simulink model "sampleModel1965_5"  (R2023a)
settings: Solver=VariableStepAuto  StartTime=0.0  StopTime=10.0  RelTol=1e-3
libraries: simulink x2, hdlsllib x2
settings Model: Creator=user1  LastModifiedBy=user1

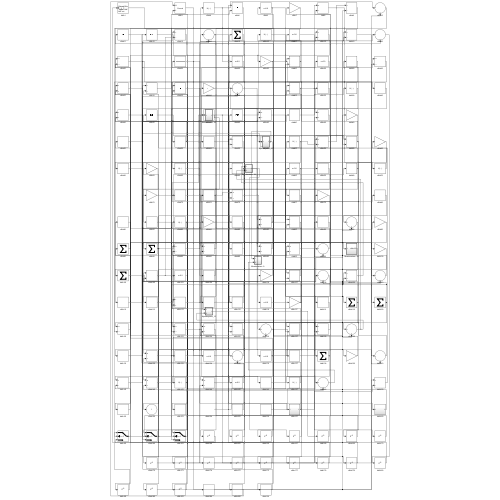
[thumbnail: Simulink's stored preview of the top-level diagram]
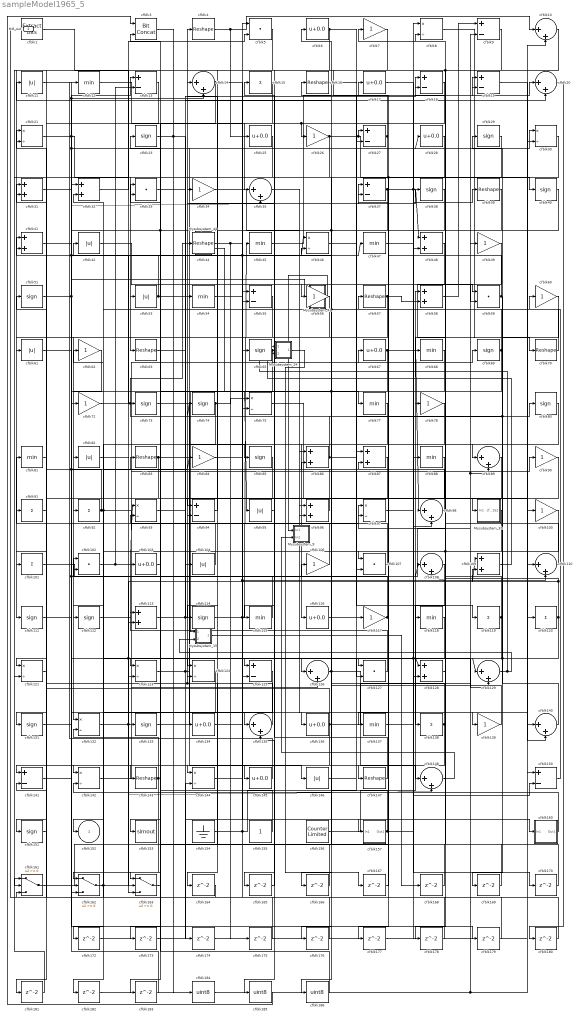
== system sampleModel1965_5 ==
  Mysubsystem_15 : Subsystem  TreatAsAtomicUnit=on  RTWFcnName=Mysubsystem_15
      settings: RTWFcnNameOpts=User specified  RTWFileNameOpts=Use function name
  Mysubsystem_24 : Subsystem  TreatAsAtomicUnit=on  RTWFcnName=Mysubsystem_24
      settings: RTWFcnNameOpts=User specified  RTWFileNameOpts=Use function name
  Mysubsystem_32 : Subsystem  TreatAsAtomicUnit=on  RTWFcnName=Mysubsystem_32
      settings: RTWFcnNameOpts=User specified  RTWFileNameOpts=Use function name
  Mysubsystem_41 : Subsystem  TreatAsAtomicUnit=on  RTWFcnName=Mysubsystem_41
      settings: RTWFcnNameOpts=User specified  RTWFileNameOpts=Use function name
  Mysubsystem_44 : Subsystem  TreatAsAtomicUnit=on  RTWFcnName=Mysubsystem_44
      settings: RTWFcnNameOpts=User specified  RTWFileNameOpts=Use function name
  Mysubsystem_9 : Subsystem  TreatAsAtomicUnit=on  RTWFcnName=Mysubsystem_9
      settings: RTWFcnNameOpts=User specified  RTWFileNameOpts=Use function name
  cfblk1 : simulink/Logic and Bit Operations/Extract Bits  bitsToExtract=Upper half  numBits=8  bitIdxRange=[0 7]  outScalingMode=Preserve fixed-point scaling
      settings: LibrarySourceBlock=|
      | hdlsllib/Logic and Bit
      | Operations/Extract Bits
  cfblk{10,14,20,35,89,98,108,110,126,129,135,140,148} (13 alike) : Sum  Inputs=|++  OutDataTypeStr=uint8
  cfblk{7,26,34,49,56,60,62,72,78,84,90,100,106,117,139} (15 alike) : Gain  OutDataTypeStr=uint8
  cfblk{15,91..92,101,119..120,138} (7 alike) : Sum  Inputs=+  OutDataTypeStr=uint8
  cfblk{5,33,59,102,107,127} (6 alike) : DotProduct  OutDataTypeStr=uint8
  cfblk{6,17,25,28,67,103,116,134,136,145} (10 alike) : Bias  Bias=0.0  SaturateOnIntegerOverflow=off
  cfblk{11,42,53,61,82,95,104,146} (8 alike) : Abs  OutDataTypeStr=uint8  SaturateOnIntegerOverflow=off
  cfblk{31..32,41,48,58,86..87,96,109,113,128} (11 alike) : Sum  OutDataTypeStr=uint8
  cfblk{23,29,38,40,51,65,69,73..74,80,85,111..112,114,131,133,151} (17 alike) : Signum
  cfblk{12,45,47,54,68,77,81,88,115,118,137} (11 alike) : MinMax  OutDataTypeStr=uint8
  cfblk{8,21,30,46,75,93,97,121,123..124,132,142,144} (13 alike) : Product  Inputs=*/  OutDataTypeStr=uint8  RndMeth=Zero  SaturateOnIntegerOverflow=on
  cfblk{9,13,18..19,27,37,55,94,125,141,150} (11 alike) : Sum  Inputs=+-  OutDataTypeStr=uint8
  cfblk{4,16,39,44,57,63,70,83,143,147} (10 alike) : Reshape
  cfblk153 : ToWorkspace  VariableName=simout  SaveFormat=Timeseries  SampleTime=-1
  cfblk154 : Ground
  cfblk155 : Constant  OutDataTypeStr=uint8  SampleTime=-1
  cfblk156 : hdlsllib/Sources/Counter Limited  uplimit=7  tsamp=-1
  cfblk157 : Subsystem
      settings: LibrarySourceBlock=|
      | hdlsllib/Ports &
      | Subsystems/Subsystem
  cfblk160 : Subsystem
      settings: LibrarySourceBlock=|
      | hdlsllib/Ports &
      | Subsystems/Subsystem
  cfblk161 : Switch  OutDataTypeStr=uint8  SaturateOnIntegerOverflow=off  InputSameDT=off
  cfblk162 : Switch  OutDataTypeStr=uint8  SaturateOnIntegerOverflow=off  InputSameDT=off
  cfblk163 : Switch  OutDataTypeStr=uint8  SaturateOnIntegerOverflow=off  InputSameDT=off
  cfblk{164..170,172..183} (19 alike) : Delay  SampleTime=1
  cfblk184 : DataTypeConversion  OutDataTypeStr=uint8  SaturateOnIntegerOverflow=off  RndMeth=Floor
  cfblk185 : DataTypeConversion  OutDataTypeStr=uint8  SaturateOnIntegerOverflow=off  RndMeth=Floor
  cfblk186 : DataTypeConversion  OutDataTypeStr=uint8  SaturateOnIntegerOverflow=off  RndMeth=Floor
  cfblk3 : hdlsllib/Logic and Bit Operations/Bit Concat  numInputs=2
  cfblk152 : Outport  OutDataTypeStr=uint8  VectorParamsAs1DForOutWhenUnconnected=off
  Hdl_out : Outport  Port=2  OutDataTypeStr=uint8
  wires:
  cfblk65/1 -> cfblk139/1, cfblk183/1
  cfblk42/1 -> cfblk56/1
  cfblk73/1 -> cfblk135/1
  cfblk77/1 -> cfblk116/1
  cfblk92/1 -> cfblk69/1, cfblk162/1, cfblk21/2
  cfblk58/1 -> cfblk9/1
  cfblk48/1 -> cfblk70/1
  cfblk53/1 -> cfblk37/1, cfblk31/2
  cfblk157/1(Out1) -> cfblk16/1, cfblk150/2
  cfblk145/1 -> cfblk12/1
  cfblk114/1 -> cfblk45/1, cfblk67/1
  cfblk150/1 -> cfblk60/1
  cfblk161/1 -> cfblk147/1
  cfblk110/1 -> cfblk7/1
  cfblk4/1 -> cfblk10/1, cfblk25/1
  cfblk112/1 -> cfblk90/1
  cfblk27/1 -> cfblk111/1, cfblk75/2
  cfblk86/1 -> Mysubsystem_44/1(In1), cfblk73/1, cfblk80/1
  cfblk14/1 -> cfblk129/2, cfblk173/1
  cfblk8/1 -> cfblk100/1
  cfblk56/1 -> cfblk132/1
  cfblk133/1 -> cfblk30/1
  cfblk118/1 -> cfblk142/1
  cfblk87/1 -> cfblk92/1
  cfblk141/1 -> cfblk47/1, cfblk35/2, cfblk84/1, cfblk108/1
  cfblk3/1 -> cfblk184/1
  cfblk115/1 -> cfblk102/1
  cfblk123/1 -> cfblk146/1, cfblk160/1(In1)
  cfblk39/1 -> cfblk115/1
  cfblk98/1 -> cfblk42/1
  cfblk35/1 -> cfblk96/1
  cfblk143/1 -> cfblk132/2, cfblk172/1
  cfblk28/1 -> cfblk126/1, cfblk177/1
  cfblk135/1 -> cfblk4/1, cfblk31/1
  cfblk19/1 -> cfblk120/1
  cfblk147/1 -> cfblk34/1
  cfblk29/1 -> cfblk63/1
  cfblk121/1 -> cfblk41/1
  cfblk75/1 -> cfblk110/1
  cfblk18/1 -> cfblk26/1, cfblk164/1
  cfblk62/1 -> cfblk82/1
  cfblk162/1 -> cfblk62/1, cfblk109/2
  cfblk156/1 -> cfblk58/1
  cfblk108/1 -> cfblk138/1
  cfblk13/1 -> cfblk101/1
  cfblk81/1 -> cfblk141/1
  cfblk101/1 -> cfblk106/1
  cfblk30/1 -> cfblk53/1
  cfblk45/1 -> cfblk19/1
  cfblk57/1 -> cfblk131/1, cfblk58/2
  cfblk132/1 -> cfblk97/1, cfblk148/2
  cfblk131/1 -> cfblk72/1
  cfblk6/1 -> cfblk119/1, cfblk163/2
  cfblk85/1 -> cfblk121/1
  cfblk74/1 -> cfblk112/1, cfblk75/1
  cfblk129/1 -> Mysubsystem_24/2(In2), Mysubsystem_15/2(In2)
  cfblk67/1 -> cfblk98/1, cfblk107/2
  cfblk21/1 -> cfblk113/2, cfblk179/1
  cfblk26/1 -> cfblk27/1, cfblk140/1, cfblk121/2
  cfblk142/1 -> cfblk126/2
  cfblk51/1 -> cfblk123/1, cfblk46/2
  cfblk70/1 -> cfblk32/2, cfblk6/1
  cfblk40/1 -> cfblk125/1
  cfblk9/1 -> cfblk61/1, cfblk178/1
  cfblk88/1 -> cfblk151/1
  cfblk11/1 -> Mysubsystem_41/1(In1), cfblk14/2
  cfblk68/1 -> cfblk95/1, cfblk166/1
  cfblk49/1 -> cfblk68/1
  cfblk128/1 -> cfblk78/1
  cfblk120/1 -> cfblk8/2, cfblk109/1, cfblk127/2
  cfblk72/1 -> cfblk44/1
  cfblk7/1 -> cfblk94/1
  cfblk10/1 -> cfblk145/1
  cfblk94/1 -> cfblk14/1
  cfblk54/1 -> cfblk59/1
  cfblk46/1 -> cfblk87/1
  cfblk83/1 -> cfblk85/1, cfblk162/2
  cfblk160/1(Out1) -> cfblk142/2
  cfblk102/1 -> cfblk93/1, cfblk13/2
  cfblk104/1 -> cfblk81/1
  cfblk78/1 -> cfblk96/2
  cfblk146/1 -> cfblk19/2
  cfblk139/1 -> cfblk41/2
  cfblk103/1 -> cfblk143/1
  cfblk17/1 -> cfblk98/2
  cfblk44/1 -> cfblk59/2, cfblk175/1
  cfblk116/1 -> cfblk117/1
  cfblk89/1 -> cfblk127/1
  cfblk138/1 -> cfblk11/1, cfblk181/1
  cfblk96/1 -> cfblk54/1
  cfblk33/1 -> cfblk104/1
  cfblk84/1 -> cfblk110/2, cfblk157/1(In1)
  cfblk137/1 -> cfblk88/1
  cfblk23/1 -> Mysubsystem_32/1(In1), cfblk134/1
  cfblk59/1 -> cfblk17/1, cfblk89/1
  cfblk5/1 -> cfblk161/2
  cfblk113/1 -> cfblk9/2, cfblk20/2
  cfblk41/1 -> cfblk136/1
  cfblk34/1 -> cfblk86/1
  cfblk126/1 -> cfblk148/1, cfblk176/1
  cfblk37/1 -> cfblk48/1, cfblk40/1, cfblk163/3
  cfblk61/1 -> cfblk28/1, cfblk13/1
  cfblk140/1 -> cfblk74/1, cfblk29/1
  cfblk80/1 -> cfblk114/1
  cfblk15/1 -> cfblk35/1
  cfblk107/1 -> cfblk94/2
  cfblk134/1 -> cfblk65/1
  cfblk119/1 -> cfblk97/2, cfblk137/1
  cfblk154/1 -> cfblk5/1, cfblk27/2
  cfblk117/1 -> cfblk23/1, cfblk87/2
  cfblk25/1 -> cfblk125/2
  cfblk69/1 -> cfblk107/1, cfblk57/1
  cfblk12/1 -> cfblk55/2
  cfblk111/1 -> cfblk83/1
  cfblk106/1 -> cfblk15/1
  cfblk127/1 -> cfblk103/1
  cfblk136/1 -> cfblk144/1, cfblk20/1, cfblk21/1
  cfblk144/1 -> cfblk38/1, cfblk46/1
  cfblk124/1 -> cfblk163/1
  cfblk1/1 -> cfblk133/1
  cfblk82/1 -> cfblk128/1, cfblk128/2, cfblk140/2
  cfblk93/1 -> cfblk18/1
  cfblk91/1 -> cfblk51/1
  cfblk100/1 -> cfblk124/1, cfblk108/2
  cfblk155/1 -> cfblk113/1
  cfblk163/1 -> cfblk33/1
  cfblk32/1 -> cfblk5/2
  cfblk55/1 -> cfblk123/2
  cfblk151/1 -> cfblk91/1
  cfblk16/1 -> cfblk118/1
  cfblk38/1 -> cfblk153/1, cfblk162/3, cfblk186/1
  cfblk31/1 -> cfblk77/1
  cfblk60/1 -> cfblk129/1, cfblk169/1
  cfblk47/1 -> cfblk39/1
  cfblk164/1 -> cfblk1/1
  cfblk95/1 -> cfblk165/1
  cfblk165/1 -> cfblk135/2
  cfblk166/1 -> cfblk93/2
  cfblk167/1 -> cfblk37/2
  cfblk168/1 -> cfblk86/2
  cfblk169/1 -> cfblk18/2
  cfblk97/1 -> cfblk170/1
  cfblk170/1 -> cfblk124/2
  cfblk172/1 -> cfblk144/2
  cfblk173/1 -> cfblk8/1
  cfblk63/1 -> cfblk174/1
  cfblk174/1 -> cfblk10/2
  cfblk175/1 -> cfblk102/2
  cfblk176/1 -> cfblk161/3
  cfblk177/1 -> cfblk48/2
  cfblk178/1 -> cfblk33/2
  cfblk179/1 -> cfblk141/2
  cfblk20/1 -> cfblk180/1
  cfblk180/1 -> cfblk55/1
  cfblk181/1 -> cfblk161/1
  cfblk125/1 -> cfblk182/1
  cfblk182/1 -> cfblk30/2
  cfblk183/1 -> cfblk32/1
  cfblk184/1 -> cfblk89/2, cfblk49/1, cfblk150/1
  cfblk90/1 -> cfblk185/1
  cfblk185/1 -> cfblk3/1
  cfblk186/1 -> cfblk3/2
  cfblk148/1 -> Mysubsystem_9/2(In2)
  Mysubsystem_15/1(Out1) -> cfblk168/1
  cfblk109/1 -> Mysubsystem_24/1(In1)
  Mysubsystem_24/1(Out1) -> cfblk167/1
  Mysubsystem_32/1(cfblk152) -> cfblk152/1
  Mysubsystem_41/1(Out1) -> Mysubsystem_9/1(In1)
  Mysubsystem_44/1(Out1) -> Mysubsystem_15/1(In1)

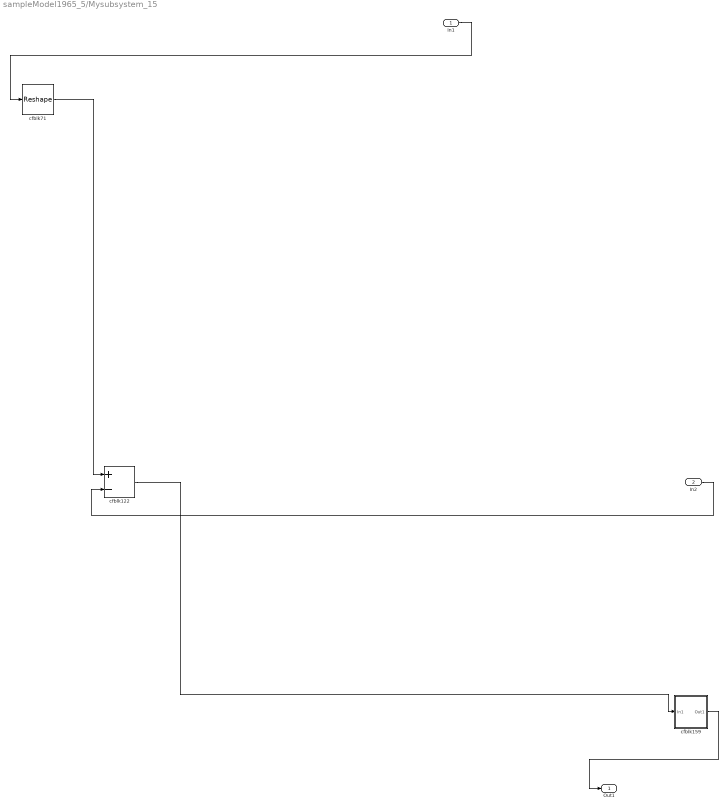
== system sampleModel1965_5/Mysubsystem_15 ==
  In1 : Inport
  In2 : Inport  Port=2
  cfblk122 : Sum  Inputs=+-
  cfblk159 : Subsystem
      settings: LibrarySourceBlock=|
      | hdlsllib/Ports &
      | Subsystems/Subsystem
  cfblk71 : Reshape
  Out1 : Outport
  wires:
  In2/1 -> cfblk122/2
  cfblk71/1 -> cfblk122/1
  cfblk159/1(Out1) -> Out1/1
  cfblk122/1 -> cfblk159/1(In1)
  In1/1 -> cfblk71/1

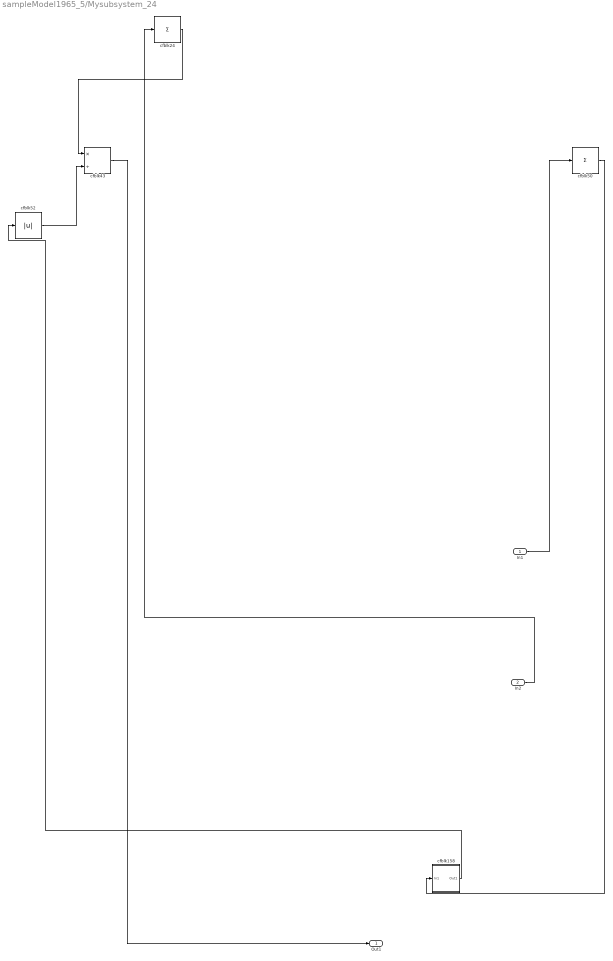
== system sampleModel1965_5/Mysubsystem_24 ==
  In1 : Inport
  In2 : Inport  Port=2
  cfblk158 : Subsystem
      settings: LibrarySourceBlock=|
      | hdlsllib/Ports &
      | Subsystems/Subsystem
  cfblk24 : Sum  Inputs=+
  cfblk43 : Product  Inputs=*/  RndMeth=Zero  SaturateOnIntegerOverflow=on
  cfblk50 : Sum  Inputs=+
  cfblk52 : Abs  SaturateOnIntegerOverflow=off
  Out1 : Outport
  wires:
  cfblk52/1 -> cfblk43/2
  cfblk50/1 -> cfblk158/1(In1)
  In1/1 -> cfblk50/1
  cfblk43/1 -> Out1/1
  cfblk158/1(Out1) -> cfblk52/1
  cfblk24/1 -> cfblk43/1
  In2/1 -> cfblk24/1

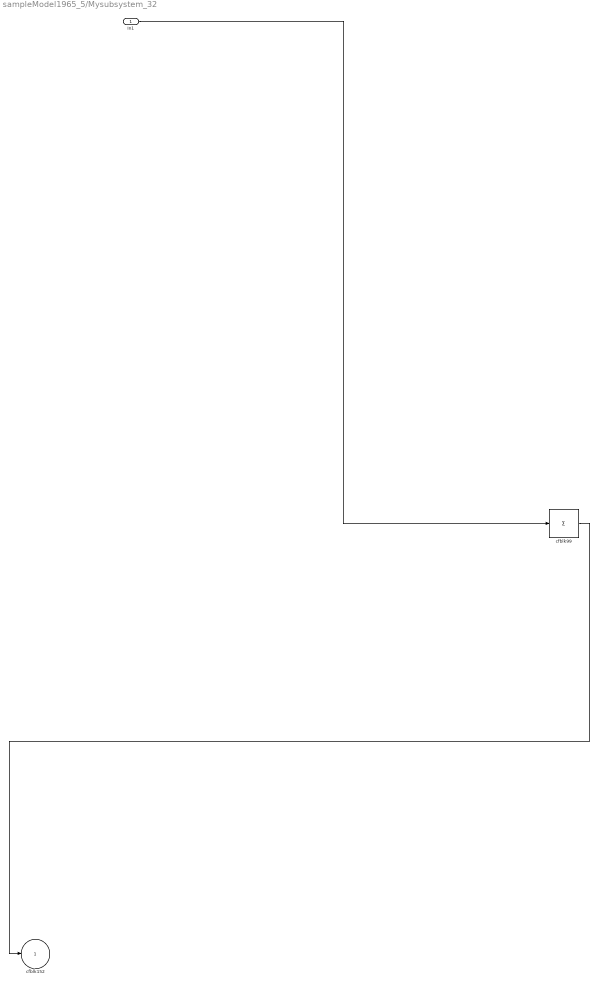
== system sampleModel1965_5/Mysubsystem_32 ==
  In1 : Inport
  cfblk99 : Sum  Inputs=+
  cfblk152 : Outport  VectorParamsAs1DForOutWhenUnconnected=off
  wires:
  cfblk99/1 -> cfblk152/1
  In1/1 -> cfblk99/1

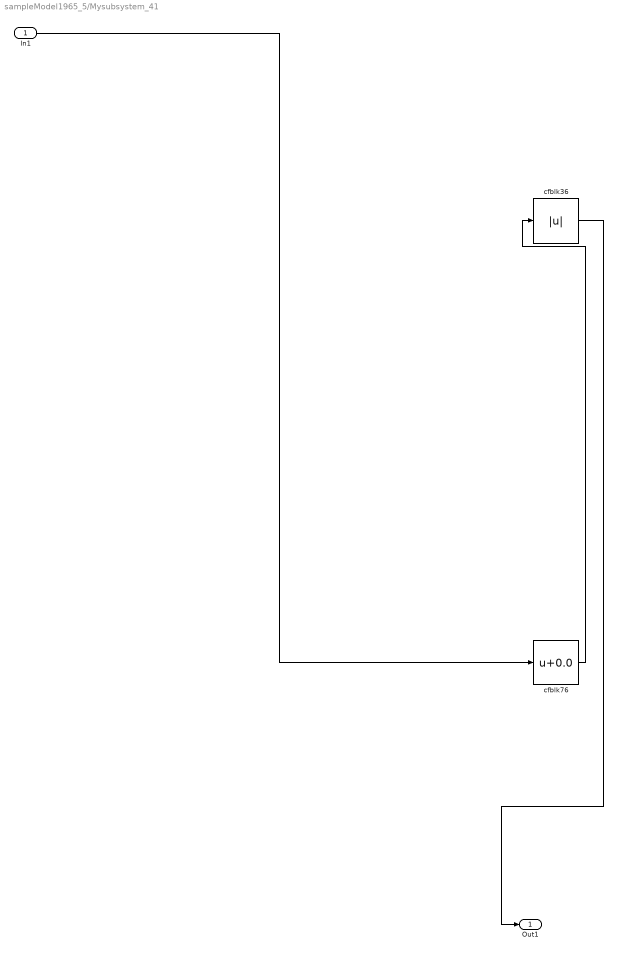
== system sampleModel1965_5/Mysubsystem_41 ==
  In1 : Inport
  cfblk36 : Abs  SaturateOnIntegerOverflow=off
  cfblk76 : Bias  Bias=0.0  SaturateOnIntegerOverflow=off
  Out1 : Outport
  wires:
  cfblk76/1 -> cfblk36/1
  In1/1 -> cfblk76/1
  cfblk36/1 -> Out1/1

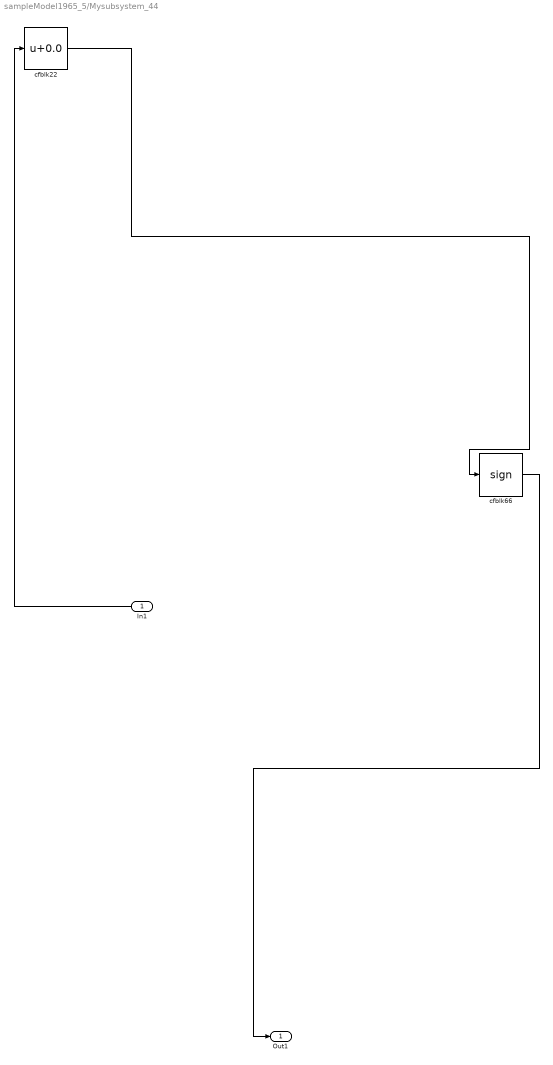
== system sampleModel1965_5/Mysubsystem_44 ==
  In1 : Inport
  cfblk22 : Bias  Bias=0.0  SaturateOnIntegerOverflow=off
  cfblk66 : Signum
  Out1 : Outport
  wires:
  cfblk22/1 -> cfblk66/1
  cfblk66/1 -> Out1/1
  In1/1 -> cfblk22/1

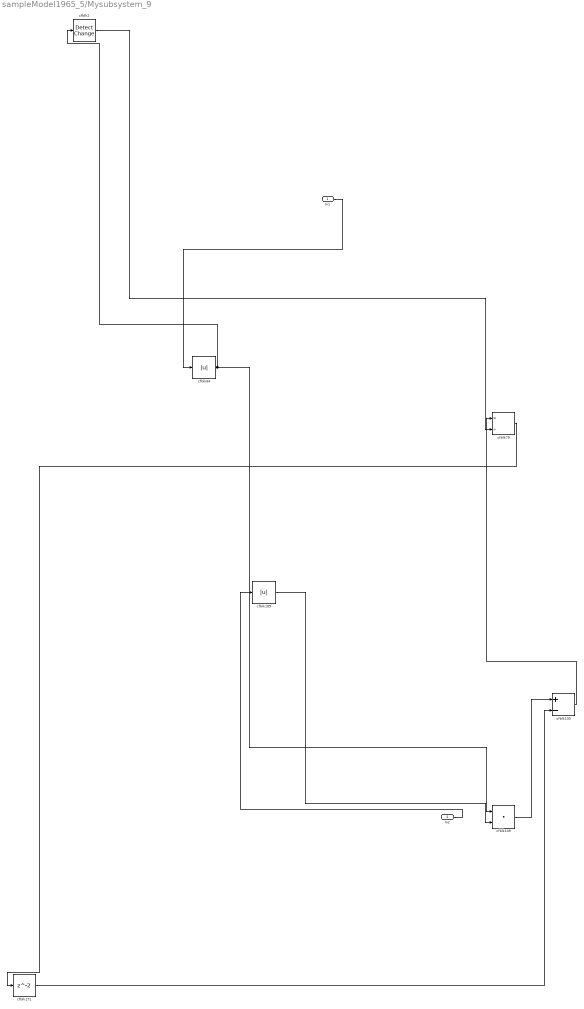
== system sampleModel1965_5/Mysubsystem_9 ==
  In1 : Inport
  In2 : Inport  Port=2
  cfblk105 : Abs  SaturateOnIntegerOverflow=off
  cfblk130 : Sum  Inputs=+-
  cfblk149 : DotProduct  OutDataTypeStr=Inherit: Inherit via internal rule
  cfblk171 : Delay  SampleTime=1
  cfblk2 : simulink/Logic and Bit Operations/Detect Change  vinit=0  OutDataTypeStr=boolean
      settings: LibrarySourceBlock=|
      | hdlsllib/Logic and Bit
      | Operations/Detect
      | Change
  cfblk64 : Abs  SaturateOnIntegerOverflow=off
  cfblk79 : Product  Inputs=*/  RndMeth=Zero  SaturateOnIntegerOverflow=on
  wires:
  cfblk79/1 -> cfblk171/1
  cfblk105/1 -> cfblk149/2
  cfblk64/1 -> cfblk149/1, cfblk2/1
  cfblk171/1 -> cfblk130/2
  In2/1 -> cfblk105/1
  cfblk130/1 -> cfblk79/1
  cfblk149/1 -> cfblk130/1
  cfblk2/1 -> cfblk79/2
  In1/1 -> cfblk64/1

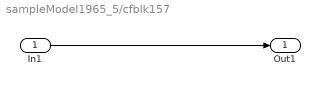
== system sampleModel1965_5/cfblk157 ==
  In1 : Inport
  Out1 : Outport
  wires:
  In1/1 -> Out1/1

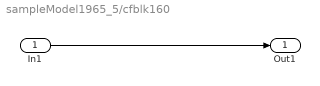
== system sampleModel1965_5/cfblk160 ==
  In1 : Inport
  Out1 : Outport
  wires:
  In1/1 -> Out1/1

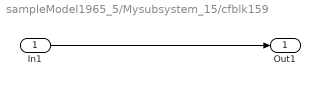
== system sampleModel1965_5/Mysubsystem_15/cfblk159 ==
  In1 : Inport
  Out1 : Outport
  wires:
  In1/1 -> Out1/1

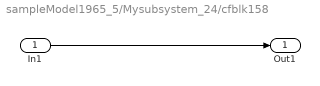
== system sampleModel1965_5/Mysubsystem_24/cfblk158 ==
  In1 : Inport
  Out1 : Outport
  wires:
  In1/1 -> Out1/1
